simulink model "Simulator_Case_8"  (R2024a)
settings: Solver=VariableStepAuto  StartTime=0.0  StopTime=1400  RelTol=1e-3
values from neighbouring files (symbols this model uses):
  Declination_Sigean = 2.116*(pi/180)    (= 0.0369311669722)    [Parametrization_Simulation_Case_8.m]
  Position_Initial_X = Waypoints_X(1)    [Parametrization_Simulation_Case_8.m]
  Position_Initial_Y = Waypoints_Y(1)    [Parametrization_Simulation_Case_8.m]
  Time_Guidance_Sampling = 20    [Parametrization_Simulation_Case_8.m]
  Time_Period_Sampling = 0.1    [Parametrization_Simulation_Case_8.m]
  Velocity_Norm_Control_Vector = 0    [Velocity_Profile_Norm_Case_8.m]
undefined symbols (not defined in the file or in its folder): Area_Lateral_Projected_Wind, Damping_Coefficient, Damping_Factor_Waves, Density_Air, Density_Water_Salted, Draft_Depth, Drag_Coefficient, Gain_Filter, Inertia_Moment, Length_Ship, Longeron_Area, Mass_Ship, Pulsation_Natural, Pulsation_Wave, Rudder_Angle_Maximal, Rudder_Angle_Minimal, Rudder_Rate_Maximal, Rudder_Rate_Minimal, Static_Gain_Nomoto, Structure_Wind_Coefficient, Time_Constant_Total, Time_Stored, Velocity_Ship_Mean, Waypoints, Yaw_Control_Hydrodynamics_Derivative
libraries: simulink_extras x7, cstblocks x2, sensorinslib x2, sensorgpslib x1
(part 1 of 2)
settings Model: Creator=gerar  LastModifiedBy=gerar

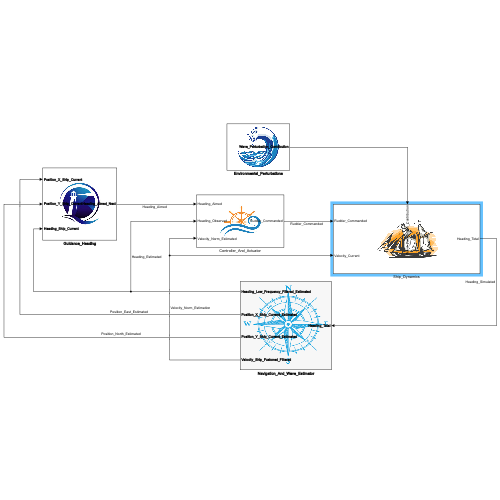
[thumbnail: Simulink's stored preview of the top-level diagram]
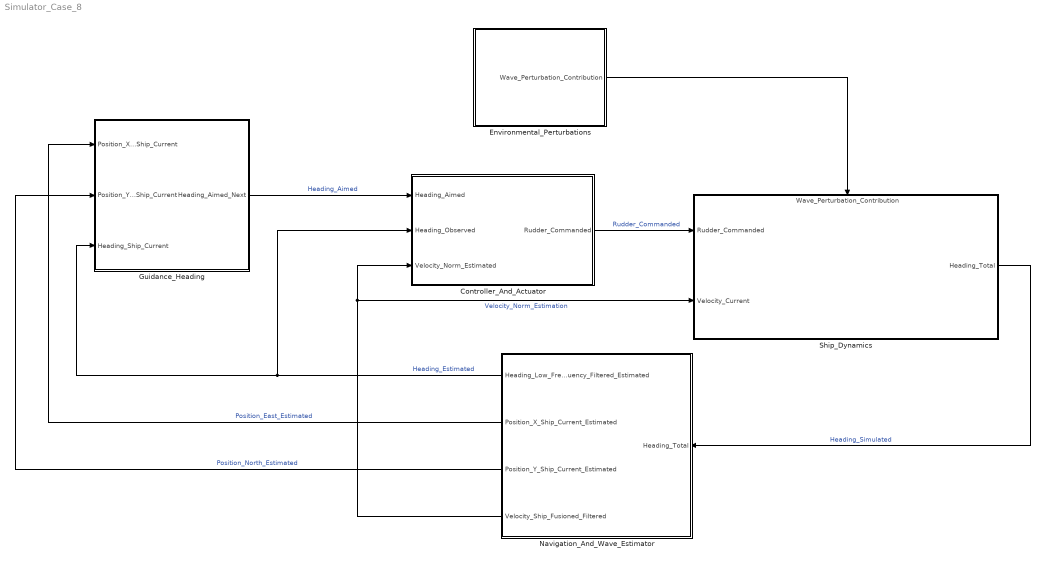
== system Simulator_Case_8 ==
  Controller_And_Actuator : Subsystem
      mask Display: image('Rudder3.jpg');
  Environmental_Perturbations : Subsystem
      mask Display: image('Wave2.png');
  Guidance_Heading : Subsystem
      mask Display: image('phare4.jpg');
  Navigation_And_Wave_Estimator : Subsystem
      mask Display: image('compass4.png');
  Ship_Dynamics : Subsystem
      settings: PortSchema="{\"entries\":[{\"content\":{\"sides\":[{\"content\":{\"connectorIds\":[\"In1\",\"In2\"]},\"type\":\"ConnectorPlacement.EquallySpacedRectSide\",\"uuid\":\"1262d93f-9737-49c5-b1c8-13d3f825160d\"},{\"content\":{\"connectorIds\":[\"Out1\"],\"side\":\"RIGHT\"},\"type\":\"ConnectorPlacement.EquallySpacedRectSide\",\"uuid\":\"2783823e-17f0-4da0-9b4a-e84aa912eb5f\"},{\"content\":{\"connectorIds\":[\"In3\"],\"side\":\"TOP\"},\"type\":\"ConnectorPlacement.EquallySpacedRectSide\",\"uuid\":\"9227960a-c500-4bd1-9392-f2e1de824969\"}]},\"type\":\"ConnectorPlacement.EquallySpacedConnector\",\"uuid\":\"fe1a7a14-057d-49da-982c-994c0d128614\"}],\"packageUris\":[\"http://schema.mathworks.com/mf0/Connector/R2020b\"],\"version\":\"1.0\"}"
      mask Display: image('ship2.png');
  wires:
  Guidance_Heading/1(Heading_Aimed_Next) -> Controller_And_Actuator/1(Heading_Aimed)  "Heading_Aimed"
  Navigation_And_Wave_Estimator/1(Heading_Low_Frequency_Filtered_Estimated) -> Controller_And_Actuator/2(Heading_Observed), Guidance_Heading/3(Heading_Ship_Current)  "Heading_Estimated"
  Environmental_Perturbations/1(Wave_Perturbation_Contribution) -> Ship_Dynamics/3(Wave_Perturbation_Contribution)
  Ship_Dynamics/1(Heading_Total) -> Navigation_And_Wave_Estimator/1(Heading_Total)  "Heading_Simulated"
  Navigation_And_Wave_Estimator/3(Position_Y_Ship_Current_Estimated) -> Guidance_Heading/2(Position_Y_Ship_Current)  "Position_North_Estimated"
  Navigation_And_Wave_Estimator/2(Position_X_Ship_Current_Estimated) -> Guidance_Heading/1(Position_X_Ship_Current)  "Position_East_Estimated"
  Controller_And_Actuator/1(Rudder_Commanded) -> Ship_Dynamics/1(Rudder_Commanded)  "Rudder_Commanded"
  Navigation_And_Wave_Estimator/4(Velocity_Ship_Fusioned_Filtered) -> Ship_Dynamics/2(Velocity_Current), Controller_And_Actuator/3(Velocity_Norm_Estimated)  "Velocity_Norm_Estimation"

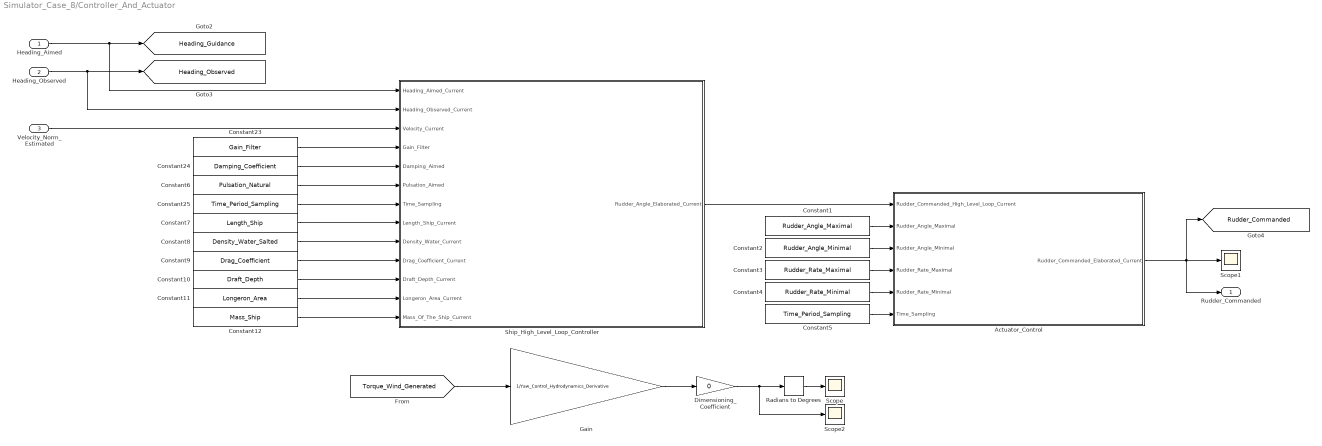
== system Simulator_Case_8/Controller_And_Actuator ==
  Heading_Aimed : Inport
  Heading_Observed : Inport  Port=2
  Velocity_Norm_Estimated : Inport  Port=3
  Actuator_Control : MATLAB Function  TreatAsAtomicUnit=on  SystemSampleTime=Time_Period_Sampling
  Constant1 : Constant  Value=Rudder_Angle_Maximal
  Constant10 : Constant  Value=Draft_Depth
  Constant11 : Constant  Value=Longeron_Area
  Constant12 : Constant  Value=Mass_Ship
  Constant2 : Constant  Value=Rudder_Angle_Minimal
  Constant23 : Constant  Value=Gain_Filter
  Constant24 : Constant  Value=Damping_Coefficient
  Constant25 : Constant  Value=Time_Period_Sampling
  Constant3 : Constant  Value=Rudder_Rate_Maximal
  Constant4 : Constant  Value=Rudder_Rate_Minimal
  Constant5 : Constant  Value=Time_Period_Sampling
  Constant6 : Constant  Value=Pulsation_Natural
  Constant7 : Constant  Value=Length_Ship
  Constant8 : Constant  Value=Density_Water_Salted
  Constant9 : Constant  Value=Drag_Coefficient
  Dimensioning_Coefficient : Gain  Gain=0
  Gain : Gain  Gain=1/Yaw_Control_Hydrodynamics_Derivative
  Radians to Degrees : simulink_extras/Transformations/Radians to Degrees
  Scope : Scope
  Scope1 : Scope
  Scope2 : Scope
  Ship_High_Level_Loop_Controller : MATLAB Function  TreatAsAtomicUnit=on  SystemSampleTime=Time_Period_Sampling
  Rudder_Commanded : Outport
  tag scope: Heading_Guidance=global, Heading_Observed=global, Rudder_Commanded=global
  wires:
  [Torque_Wind_Generated] -> Gain/1
  Gain/1 -> Dimensioning_Coefficient/1
  Radians to Degrees/1 -> Scope/1
  Dimensioning_Coefficient/1 -> Scope2/1, Radians to Degrees/1
  Heading_Aimed/1 -> [Heading_Guidance], Ship_High_Level_Loop_Controller/1(Heading_Aimed_Current)
  Heading_Observed/1 -> Ship_High_Level_Loop_Controller/2(Heading_Observed_Current), [Heading_Observed]
  Ship_High_Level_Loop_Controller/1(Rudder_Angle_Elaborated_Current) -> Actuator_Control/1(Rudder_Commanded_High_Level_Loop_Current)
  Constant1/1 -> Actuator_Control/2(Rudder_Angle_Maximal)
  Constant2/1 -> Actuator_Control/3(Rudder_Angle_Minimal)
  Constant3/1 -> Actuator_Control/4(Rudder_Rate_Maximal)
  Constant4/1 -> Actuator_Control/5(Rudder_Rate_Minimal)
  Constant5/1 -> Actuator_Control/6(Time_Sampling)
  Actuator_Control/1(Rudder_Commanded_Elaborated_Current) -> Rudder_Commanded/1, [Rudder_Commanded], Scope1/1
  Constant23/1 -> Ship_High_Level_Loop_Controller/4(Gain_Filter)
  Constant24/1 -> Ship_High_Level_Loop_Controller/5(Damping_Aimed)
  Constant25/1 -> Ship_High_Level_Loop_Controller/7(Time_Sampling)
  Constant6/1 -> Ship_High_Level_Loop_Controller/6(Pulsation_Aimed)
  Constant7/1 -> Ship_High_Level_Loop_Controller/8(Length_Ship_Current)
  Constant8/1 -> Ship_High_Level_Loop_Controller/9(Density_Water_Current)
  Constant9/1 -> Ship_High_Level_Loop_Controller/10(Drag_Coefficient_Current)
  Constant10/1 -> Ship_High_Level_Loop_Controller/11(Draft_Depth_Current)
  Constant11/1 -> Ship_High_Level_Loop_Controller/12(Longeron_Area_Current)
  Constant12/1 -> Ship_High_Level_Loop_Controller/13(Mass_Of_The_Ship_Current)
  Velocity_Norm_Estimated/1 -> Ship_High_Level_Loop_Controller/3(Velocity_Current)

== system Simulator_Case_8/Environmental_Perturbations ==
  Gain1 : Gain  Gain=0
  Scope : Scope
  Wave-Induced_Perturbation_Motion : Subsystem
  Wind_Perturbation_Torque : Subsystem
  Wave_Perturbation_Contribution : Outport
  tag scope: Torque_Wind_Generated=global, Wave_Generated_Signal=global
  wires:
  Wave-Induced_Perturbation_Motion/1(Wave_Induced_Heading) -> Scope/1, [Wave_Generated_Signal], Wave_Perturbation_Contribution/1
  Wind_Perturbation_Torque/1(Torque_Wind) -> Gain1/1
  Gain1/1 -> [Torque_Wind_Generated]

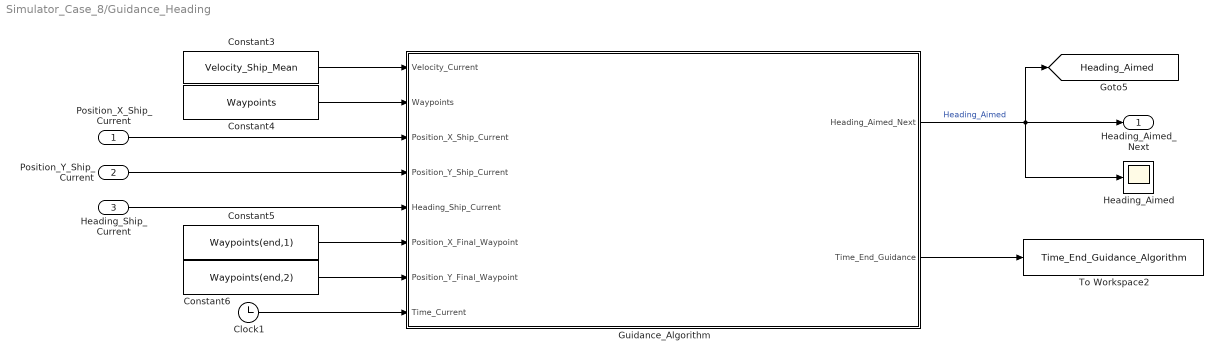
== system Simulator_Case_8/Guidance_Heading ==
  Position_X_Ship_Current : Inport
  Position_Y_Ship_Current : Inport  Port=2
  Heading_Ship_Current : Inport  Port=3
  Clock1 : Clock
  Constant3 : Constant  Value=Velocity_Ship_Mean
  Constant4 : Constant  Value=Waypoints
  Constant5 : Constant  Value=Waypoints(end,1)
  Constant6 : Constant  Value=Waypoints(end,2)
  Guidance_Algorithm : MATLAB Function  TreatAsAtomicUnit=on  SystemSampleTime=Time_Guidance_Sampling*3
  Heading_Aimed : Scope
  To Workspace2 : ToWorkspace  VariableName=Time_End_Guidance_Algorithm  SaveFormat=Timeseries  SampleTime=-1
  Heading_Aimed_Next : Outport
  tag scope: Heading_Aimed=global
  wires:
  Constant5/1 -> Guidance_Algorithm/6(Position_X_Final_Waypoint)
  Guidance_Algorithm/2(Time_End_Guidance) -> To Workspace2/1
  Constant3/1 -> Guidance_Algorithm/1(Velocity_Current)
  Position_Y_Ship_Current/1 -> Guidance_Algorithm/4(Position_Y_Ship_Current)
  Constant4/1 -> Guidance_Algorithm/2(Waypoints)
  Clock1/1 -> Guidance_Algorithm/8(Time_Current)
  Constant6/1 -> Guidance_Algorithm/7(Position_Y_Final_Waypoint)
  Position_X_Ship_Current/1 -> Guidance_Algorithm/3(Position_X_Ship_Current)
  Heading_Ship_Current/1 -> Guidance_Algorithm/5(Heading_Ship_Current)
  Guidance_Algorithm/1(Heading_Aimed_Next) -> Heading_Aimed/1, Heading_Aimed_Next/1, [Heading_Aimed]  "Heading_Aimed"

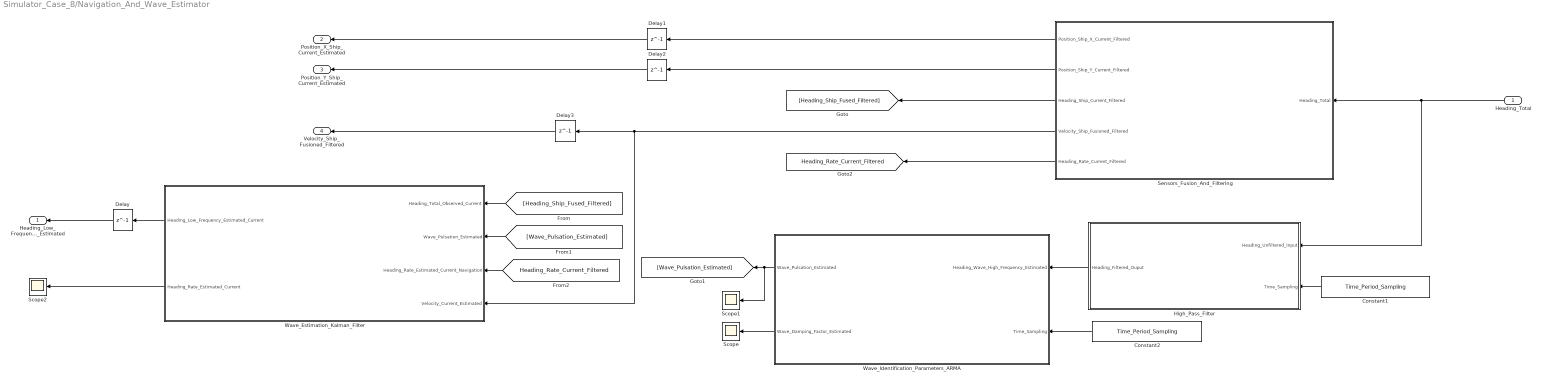
== system Simulator_Case_8/Navigation_And_Wave_Estimator ==
  Heading_Total : Inport
  Constant1 : Constant  Value=Time_Period_Sampling
  Constant2 : Constant  Value=Time_Period_Sampling
  Delay{,1..3} (4 alike) : Delay  DelayLength=1  InputProcessing=Columns as channels (frame based)  SampleTime=Time_Period_Sampling
  High_Pass_Filter : MATLAB Function  TreatAsAtomicUnit=on  SystemSampleTime=Time_Period_Sampling
  Scope : Scope
  Scope1 : Scope
  Scope2 : Scope
  Sensors_Fusion_And_Filtering : Subsystem
  Wave_Estimation_Kalman_Filter : Subsystem
  Wave_Identification_Parameters_ARMA : MATLAB Function  TreatAsAtomicUnit=on  SystemSampleTime=Time_Period_Sampling
  Heading_Low_Frequency_Filtered_Estimated : Outport
  Position_X_Ship_Current_Estimated : Outport  Port=2
  Position_Y_Ship_Current_Estimated : Outport  Port=3
  Velocity_Ship_Fusioned_Filtered : Outport  Port=4
  tag scope: Heading_Rate_Current_Filtered=global
  wires:
  Delay1/1 -> Position_X_Ship_Current_Estimated/1
  Delay2/1 -> Position_Y_Ship_Current_Estimated/1
  Sensors_Fusion_And_Filtering/1(Position_Ship_X_Current_Filtered) -> Delay1/1
  Sensors_Fusion_And_Filtering/2(Position_Ship_Y_Current_Filtered) -> Delay2/1
  Wave_Estimation_Kalman_Filter/1(Heading_Low_Frequency_Estimated_Current) -> Delay/1
  High_Pass_Filter/1(Heading_Filtered_Ouput) -> Wave_Identification_Parameters_ARMA/1(Heading_Wave_High_Frequency_Estimated)
  Constant1/1 -> High_Pass_Filter/2(Time_Sampling)
  Heading_Total/1 -> High_Pass_Filter/1(Heading_Unfiltered_Input), Sensors_Fusion_And_Filtering/1(Heading_Total)
  Delay/1 -> Heading_Low_Frequency_Filtered_Estimated/1
  Wave_Estimation_Kalman_Filter/2(Heading_Rate_Estimated_Current) -> Scope2/1
  Constant2/1 -> Wave_Identification_Parameters_ARMA/2(Time_Sampling)
  Sensors_Fusion_And_Filtering/3(Heading_Ship_Current_Filtered) -> [Heading_Ship_Fused_Filtered]
  [Heading_Ship_Fused_Filtered] -> Wave_Estimation_Kalman_Filter/1(Heading_Total_Observed_Current)
  Wave_Identification_Parameters_ARMA/1(Wave_Pulsation_Estimated) -> Scope1/1, [Wave_Pulsation_Estimated]
  [Wave_Pulsation_Estimated] -> Wave_Estimation_Kalman_Filter/2(Wave_Pulsation_Estimated)
  Wave_Identification_Parameters_ARMA/2(Wave_Damping_Factor_Estimated) -> Scope/1
  Sensors_Fusion_And_Filtering/4(Velocity_Ship_Fusioned_Filtered) -> Wave_Estimation_Kalman_Filter/4(Velocity_Current_Estimated), Delay3/1
  Delay3/1 -> Velocity_Ship_Fusioned_Filtered/1
  Sensors_Fusion_And_Filtering/5(Heading_Rate_Current_Filtered) -> [Heading_Rate_Current_Filtered]
  [Heading_Rate_Current_Filtered] -> Wave_Estimation_Kalman_Filter/3(Heading_Rate_Estimated_Current_Navigation)

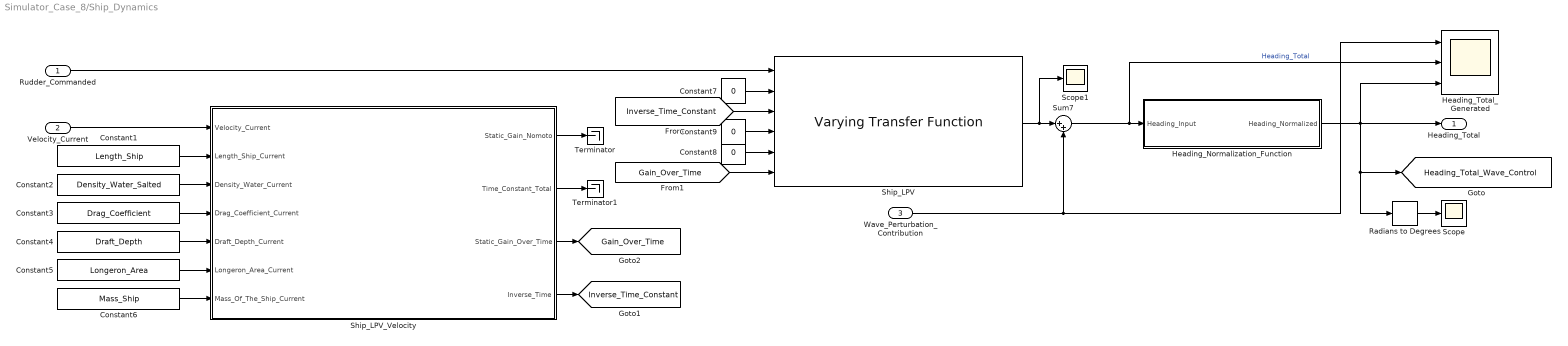
== system Simulator_Case_8/Ship_Dynamics ==
  Rudder_Commanded : Inport
  Velocity_Current : Inport  Port=2
  Wave_Perturbation_Contribution : Inport  Port=3
  Constant1 : Constant  Value=Length_Ship
  Constant2 : Constant  Value=Density_Water_Salted
  Constant3 : Constant  Value=Drag_Coefficient
  Constant4 : Constant  Value=Draft_Depth
  Constant5 : Constant  Value=Longeron_Area
  Constant6 : Constant  Value=Mass_Ship
  Constant7 : Constant  Value=0
  Constant8 : Constant  Value=0
  Constant9 : Constant  Value=0
  Heading_Normalization_Function : MATLAB Function  TreatAsAtomicUnit=on
  Heading_Total_Generated : Scope  NumInputPorts=3
  Radians to Degrees : simulink_extras/Transformations/Radians to Degrees
  Scope : Scope
  Scope1 : Scope
  Ship_LPV : cstblocks/Linear Parameter Varying/Varying Transfer Function  N=2  Feedthrough=on
  Ship_LPV_Velocity : MATLAB Function  TreatAsAtomicUnit=on
  Sum7 : Sum  Inputs=|++
  Terminator : Terminator
  Terminator1 : Terminator
  Heading_Total : Outport
  tag scope: Gain_Over_Time=global, Heading_Total_Wave_Control=global, Inverse_Time_Constant=global
  wires:
  Ship_LPV/1 -> Scope1/1, Sum7/1
  Wave_Perturbation_Contribution/1 -> Sum7/2, Heading_Total_Generated/1
  Sum7/1 -> Heading_Total_Generated/2, Heading_Normalization_Function/1(Heading_Input)  "Heading_Total"
  Radians to Degrees/1 -> Scope/1
  Heading_Normalization_Function/1(Heading_Normalized) -> Radians to Degrees/1, [Heading_Total_Wave_Control], Heading_Total_Generated/3, Heading_Total/1
  Constant1/1 -> Ship_LPV_Velocity/2(Length_Ship_Current)
  Constant3/1 -> Ship_LPV_Velocity/4(Drag_Coefficient_Current)
  Constant6/1 -> Ship_LPV_Velocity/7(Mass_Of_The_Ship_Current)
  Constant4/1 -> Ship_LPV_Velocity/5(Draft_Depth_Current)
  Constant2/1 -> Ship_LPV_Velocity/3(Density_Water_Current)
  Velocity_Current/1 -> Ship_LPV_Velocity/1(Velocity_Current)
  Constant5/1 -> Ship_LPV_Velocity/6(Longeron_Area_Current)
  Constant7/1 -> Ship_LPV/2
  Constant9/1 -> Ship_LPV/4
  Constant8/1 -> Ship_LPV/5
  Rudder_Commanded/1 -> Ship_LPV/1
  Ship_LPV_Velocity/4(Inverse_Time) -> [Inverse_Time_Constant]
  [Inverse_Time_Constant] -> Ship_LPV/3
  Ship_LPV_Velocity/3(Static_Gain_Over_Time) -> [Gain_Over_Time]
  [Gain_Over_Time] -> Ship_LPV/6
  Ship_LPV_Velocity/1(Static_Gain_Nomoto) -> Terminator/1
  Ship_LPV_Velocity/2(Time_Constant_Total) -> Terminator1/1

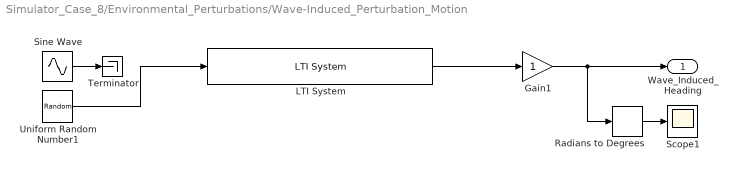
== system Simulator_Case_8/Environmental_Perturbations/Wave-Induced_Perturbation_Motion ==
  Gain1 : Gain
  LTI System : cstblocks/LTI System  sys=Wave_Transfer_Function  IC=[]  PadeOrder=0
  Radians to Degrees : simulink_extras/Transformations/Radians to Degrees
  Scope1 : Scope
  Sine Wave : Sin  Amplitude=2*(pi/180)  Frequency=Pulsation_Wave  SampleTime=0
  Terminator : Terminator
  Uniform Random Number1 : UniformRandomNumber  Minimum=-10*(pi/180)  Maximum=10*(pi/180)  SampleTime=Time_Period_Sampling
  Wave_Induced_Heading : Outport
  wires:
  Radians to Degrees/1 -> Scope1/1
  LTI System/1 -> Gain1/1
  Gain1/1 -> Radians to Degrees/1, Wave_Induced_Heading/1
  Uniform Random Number1/1 -> LTI System/1
  Sine Wave/1 -> Terminator/1

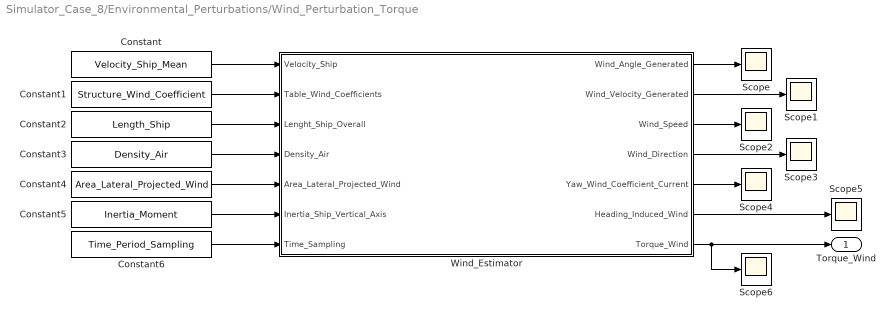
== system Simulator_Case_8/Environmental_Perturbations/Wind_Perturbation_Torque ==
  Constant : Constant  Value=Velocity_Ship_Mean
  Constant1 : Constant  Value=Structure_Wind_Coefficient
  Constant2 : Constant  Value=Length_Ship
  Constant3 : Constant  Value=Density_Air
  Constant4 : Constant  Value=Area_Lateral_Projected_Wind
  Constant5 : Constant  Value=Inertia_Moment
  Constant6 : Constant  Value=Time_Period_Sampling
  Scope{,1..6} (7 alike) : Scope
  Wind_Estimator : MATLAB Function  TreatAsAtomicUnit=on  SystemSampleTime=Time_Period_Sampling
  Torque_Wind : Outport
  wires:
  Wind_Estimator/5(Yaw_Wind_Coefficient_Current) -> Scope4/1
  Constant2/1 -> Wind_Estimator/3(Lenght_Ship_Overall)
  Constant/1 -> Wind_Estimator/1(Velocity_Ship)
  Constant5/1 -> Wind_Estimator/6(Inertia_Ship_Vertical_Axis)
  Constant4/1 -> Wind_Estimator/5(Area_Lateral_Projected_Wind)
  Constant3/1 -> Wind_Estimator/4(Density_Air)
  Wind_Estimator/1(Wind_Angle_Generated) -> Scope/1
  Wind_Estimator/2(Wind_Velocity_Generated) -> Scope1/1
  Wind_Estimator/3(Wind_Speed) -> Scope2/1
  Wind_Estimator/7(Torque_Wind) -> Torque_Wind/1, Scope6/1
  Constant1/1 -> Wind_Estimator/2(Table_Wind_Coefficients)
  Constant6/1 -> Wind_Estimator/7(Time_Sampling)
  Wind_Estimator/6(Heading_Induced_Wind) -> Scope5/1
  Wind_Estimator/4(Wind_Direction) -> Scope3/1

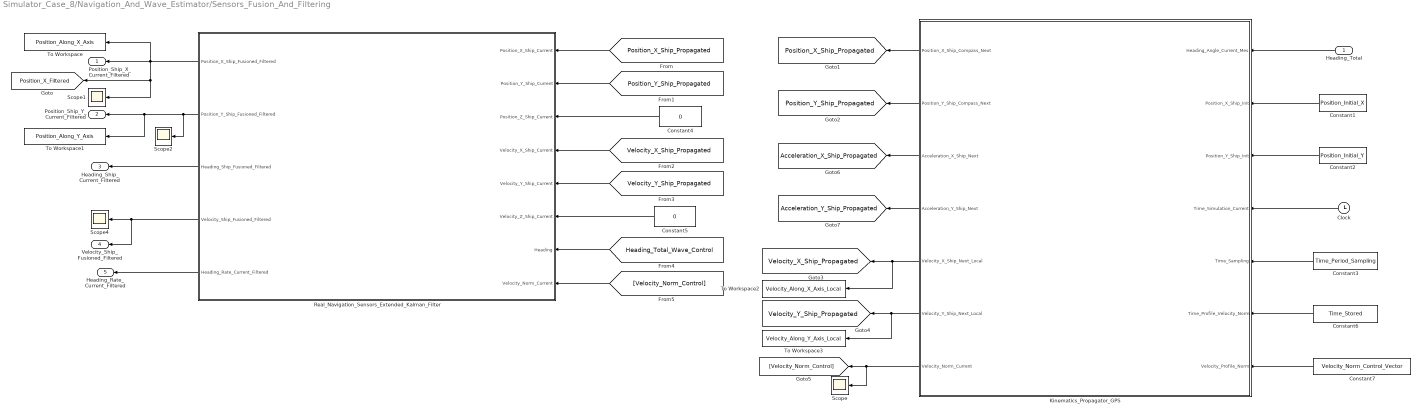
== system Simulator_Case_8/Navigation_And_Wave_Estimator/Sensors_Fusion_And_Filtering ==
  Heading_Total : Inport
  Clock : Clock
  Constant1 : Constant  Value=Position_Initial_X
  Constant2 : Constant  Value=Position_Initial_Y
  Constant3 : Constant  Value=Time_Period_Sampling
  Constant4 : Constant  Value=0
  Constant5 : Constant  Value=0
  Constant6 : Constant  Value=Time_Stored
  Constant7 : Constant  Value=Velocity_Norm_Control_Vector
  Kinematics_Propagator_GPS : MATLAB Function  TreatAsAtomicUnit=on  SystemSampleTime=Time_Period_Sampling
  Real_Navigation_Sensors_Extended_Kalman_Filter : Subsystem
  Scope{,1..2,4} (4 alike) : Scope
  To Workspace : ToWorkspace  VariableName=Position_Along_X_Axis  SaveFormat=Timeseries  SampleTime=Time_Period_Sampling
  To Workspace1 : ToWorkspace  VariableName=Position_Along_Y_Axis  SaveFormat=Timeseries  SampleTime=Time_Period_Sampling
  To Workspace2 : ToWorkspace  VariableName=Velocity_Along_X_Axis_Local  SaveFormat=Timeseries  SampleTime=Time_Period_Sampling
  To Workspace3 : ToWorkspace  VariableName=Velocity_Along_Y_Axis_Local  SaveFormat=Timeseries  SampleTime=Time_Period_Sampling
  Position_Ship_X_Current_Filtered : Outport
  Position_Ship_Y_Current_Filtered : Outport  Port=2
  Heading_Ship_Current_Filtered : Outport  Port=3
  Velocity_Ship_Fusioned_Filtered : Outport  Port=4
  Heading_Rate_Current_Filtered : Outport  Port=5
  tag scope: Acceleration_X_Ship_Propagated=global, Acceleration_Y_Ship_Propagated=global, Position_X_Filtered=global, Position_X_Ship_Propagated=global, Position_Y_Ship_Propagated=global, Velocity_X_Ship_Propagated=global, Velocity_Y_Ship_Propagated=global
  wires:
  Constant2/1 -> Kinematics_Propagator_GPS/3(Position_Y_Ship_Init)
  Clock/1 -> Kinematics_Propagator_GPS/4(Time_Simulation_Current)
  Constant1/1 -> Kinematics_Propagator_GPS/2(Position_X_Ship_Init)
  Constant3/1 -> Kinematics_Propagator_GPS/5(Time_Sampling)
  Kinematics_Propagator_GPS/3(Acceleration_X_Ship_Next) -> [Acceleration_X_Ship_Propagated]
  Kinematics_Propagator_GPS/4(Acceleration_Y_Ship_Next) -> [Acceleration_Y_Ship_Propagated]
  Heading_Total/1 -> Kinematics_Propagator_GPS/1(Heading_Angle_Current_Mes)
  Kinematics_Propagator_GPS/5(Velocity_X_Ship_Next_Local) -> To Workspace2/1, [Velocity_X_Ship_Propagated]
  Kinematics_Propagator_GPS/6(Velocity_Y_Ship_Next_Local) -> To Workspace3/1, [Velocity_Y_Ship_Propagated]
  Kinematics_Propagator_GPS/1(Position_X_Ship_Compass_Next) -> [Position_X_Ship_Propagated]
  Kinematics_Propagator_GPS/2(Position_Y_Ship_Compass_Next) -> [Position_Y_Ship_Propagated]
  [Position_X_Ship_Propagated] -> Real_Navigation_Sensors_Extended_Kalman_Filter/1(Position_X_Ship_Current)
  [Position_Y_Ship_Propagated] -> Real_Navigation_Sensors_Extended_Kalman_Filter/2(Position_Y_Ship_Current)
  Constant4/1 -> Real_Navigation_Sensors_Extended_Kalman_Filter/3(Position_Z_Ship_Current)
  [Velocity_X_Ship_Propagated] -> Real_Navigation_Sensors_Extended_Kalman_Filter/4(Velocity_X_Ship_Current)
  [Velocity_Y_Ship_Propagated] -> Real_Navigation_Sensors_Extended_Kalman_Filter/5(Velocity_Y_Ship_Current)
  Constant5/1 -> Real_Navigation_Sensors_Extended_Kalman_Filter/6(Velocity_Z_Ship_Current)
  [Heading_Total_Wave_Control] -> Real_Navigation_Sensors_Extended_Kalman_Filter/7(Heading)
  Real_Navigation_Sensors_Extended_Kalman_Filter/1(Position_X_Ship_Fusioned_Filtered) -> Scope1/1, [Position_X_Filtered], Position_Ship_X_Current_Filtered/1, To Workspace/1
  Real_Navigation_Sensors_Extended_Kalman_Filter/2(Position_Y_Ship_Fusioned_Filtered) -> Scope2/1, To Workspace1/1, Position_Ship_Y_Current_Filtered/1
  Real_Navigation_Sensors_Extended_Kalman_Filter/3(Heading_Ship_Fusioned_Filtered) -> Heading_Ship_Current_Filtered/1
  Real_Navigation_Sensors_Extended_Kalman_Filter/4(Velocity_Ship_Fusioned_Filtered) -> Velocity_Ship_Fusioned_Filtered/1, Scope4/1
  Kinematics_Propagator_GPS/7(Velocity_Norm_Current) -> Scope/1, [Velocity_Norm_Control]
  Constant6/1 -> Kinematics_Propagator_GPS/6(Time_Profile_Velocity_Norm)
  Constant7/1 -> Kinematics_Propagator_GPS/7(Velocity_Profile_Norm)
  [Velocity_Norm_Control] -> Real_Navigation_Sensors_Extended_Kalman_Filter/8(Velocity_Norm_Current)
  Real_Navigation_Sensors_Extended_Kalman_Filter/5(Heading_Rate_Current_Filtered) -> Heading_Rate_Current_Filtered/1

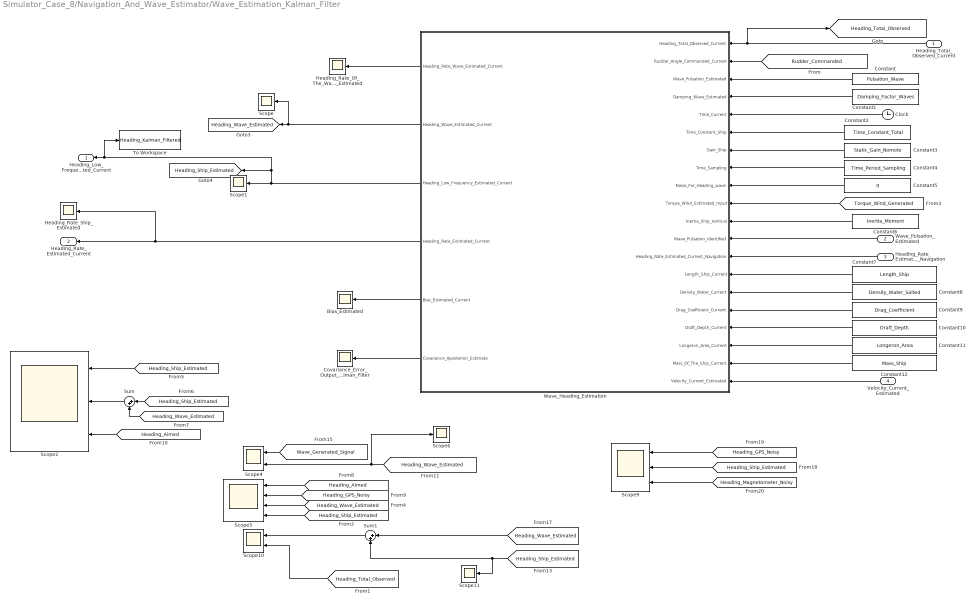
== system Simulator_Case_8/Navigation_And_Wave_Estimator/Wave_Estimation_Kalman_Filter ==
  Heading_Total_Observed_Current : Inport
  Wave_Pulsation_Estimated : Inport  Port=2
  Heading_Rate_Estimated_Current_Navigation : Inport  Port=3
  Velocity_Current_Estimated : Inport  Port=4
  Bias_Estimated : Scope
  Clock : Clock
  Constant : Constant  Value=Pulsation_Wave  SampleTime=Time_Period_Sampling
  Constant1 : Constant  Value=Damping_Factor_Waves  SampleTime=Time_Period_Sampling
  Constant10 : Constant  Value=Draft_Depth
  Constant11 : Constant  Value=Longeron_Area
  Constant12 : Constant  Value=Mass_Ship
  Constant2 : Constant  Value=Time_Constant_Total  SampleTime=Time_Period_Sampling
  Constant3 : Constant  Value=Static_Gain_Nomoto  SampleTime=Time_Period_Sampling
  Constant4 : Constant  Value=Time_Period_Sampling  SampleTime=Time_Period_Sampling
  Constant5 : Constant  Value=0
  Constant6 : Constant  Value=Inertia_Moment
  Constant7 : Constant  Value=Length_Ship
  Constant8 : Constant  Value=Density_Water_Salted
  Constant9 : Constant  Value=Drag_Coefficient
  Covariance_Error_Output_Kalman_Filter : Scope
  Heading_Rate_Of_The_Waves_Estimated : Scope
  Heading_Rate_Ship_Estimated : Scope
  Scope{,1,6,11} (4 alike) : Scope
  Scope10 : Scope  NumInputPorts=2
  Scope2 : Scope  NumInputPorts=3
  Scope4 : Scope  NumInputPorts=2
  Scope5 : Scope  NumInputPorts=4
  Scope9 : Scope  NumInputPorts=3
  Sum : Sum  Inputs=|++
  Sum1 : Sum  Inputs=|++
  To Workspace : ToWorkspace  VariableName=Heading_Kalman_Filtered  SaveFormat=Timeseries  SampleTime=Time_Period_Sampling
  Wave_Heading_Estimation : MATLAB Function  TreatAsAtomicUnit=on  SystemSampleTime=Time_Period_Sampling
  Heading_Low_Frequency_Estimated_Current : Outport
  Heading_Rate_Estimated_Current : Outport  Port=2
  tag scope: Heading_Ship_Estimated=global, Heading_Total_Observed=global, Heading_Wave_Estimated=global
  wires:
  Wave_Heading_Estimation/3(Heading_Low_Frequency_Estimated_Current) -> To Workspace/1, Heading_Low_Frequency_Estimated_Current/1, [Heading_Ship_Estimated], Scope1/1
  Heading_Total_Observed_Current/1 -> [Heading_Total_Observed], Wave_Heading_Estimation/1(Heading_Total_Observed_Current)
  [Rudder_Commanded] -> Wave_Heading_Estimation/2(Rudder_Angle_Commanded_Current)
  Constant/1 -> Wave_Heading_Estimation/3(Wave_Pulsation_Estimated)
  Constant1/1 -> Wave_Heading_Estimation/4(Damping_Wave_Estimated)
  Clock/1 -> Wave_Heading_Estimation/5(Time_Current)
  Constant2/1 -> Wave_Heading_Estimation/6(Time_Constant_Ship)
  Constant3/1 -> Wave_Heading_Estimation/7(Gain_Ship)
  Constant4/1 -> Wave_Heading_Estimation/8(Time_Sampling)
  Constant5/1 -> Wave_Heading_Estimation/9(Noise_For_Heading_wave)
  Wave_Heading_Estimation/1(Heading_Rate_Wave_Estimated_Current) -> Heading_Rate_Of_The_Waves_Estimated/1
  Wave_Heading_Estimation/2(Heading_Wave_Estimated_Current) -> Scope/1, [Heading_Wave_Estimated]
  Wave_Heading_Estimation/5(Bias_Estimated_Current) -> Bias_Estimated/1
  Wave_Heading_Estimation/4(Heading_Rate_Estimated_Current) -> Heading_Rate_Ship_Estimated/1, Heading_Rate_Estimated_Current/1
  Wave_Heading_Estimation/6(Covariance_Aposteriori_Estimate) -> Covariance_Error_Output_Kalman_Filter/1
  [Heading_Aimed] -> Scope5/1
  [Wave_Generated_Signal] -> Scope4/1
  [Heading_Ship_Estimated] -> Scope9/2
  [Heading_Magnetometer_Noisy] -> Scope9/3
  [Heading_Ship_Estimated] -> Scope11/1, Sum1/2
  [Heading_GPS_Noisy] -> Scope9/1
  [Heading_Wave_Estimated] -> Sum1/1
  Sum1/1 -> Scope10/1
  [Heading_GPS_Noisy] -> Scope5/2
  [Heading_Ship_Estimated] -> Scope5/4
  [Heading_Wave_Estimated] -> Scope6/1, Scope4/2
  [Heading_Total_Observed] -> Scope10/2
  Constant6/1 -> Wave_Heading_Estimation/11(Inertia_Ship_Vertical)
  [Torque_Wind_Generated] -> Wave_Heading_Estimation/10(Torque_Wind_Estimated_Input)
  Wave_Pulsation_Estimated/1 -> Wave_Heading_Estimation/12(Wave_Pulsation_Identified)
  Heading_Rate_Estimated_Current_Navigation/1 -> Wave_Heading_Estimation/13(Heading_Rate_Estimated_Current_Navigation)
  Constant7/1 -> Wave_Heading_Estimation/14(Length_Ship_Current)
  Constant8/1 -> Wave_Heading_Estimation/15(Density_Water_Current)
  [Heading_Wave_Estimated] -> Scope5/3
  [Heading_Ship_Estimated] -> Scope2/1
  Sum/1 -> Scope2/2
  [Heading_Ship_Estimated] -> Sum/1
  [Heading_Wave_Estimated] -> Sum/2
  [Heading_Aimed] -> Scope2/3
  Constant9/1 -> Wave_Heading_Estimation/16(Drag_Coefficient_Current)
  Constant10/1 -> Wave_Heading_Estimation/17(Draft_Depth_Current)
  Constant11/1 -> Wave_Heading_Estimation/18(Longeron_Area_Current)
  Constant12/1 -> Wave_Heading_Estimation/19(Mass_Of_The_Ship_Current)
  Velocity_Current_Estimated/1 -> Wave_Heading_Estimation/20(Velocity_Current_Estimated)

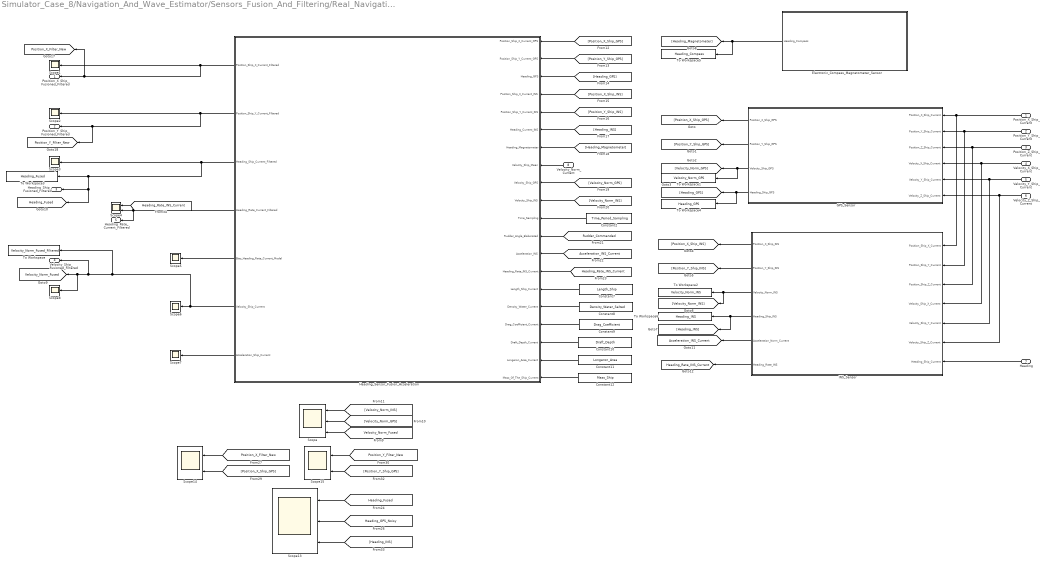
== system Simulator_Case_8/Navigation_And_Wave_Estimator/Sensors_Fusion_And_Filtering/Real_Navigation_Sensors_Extended_Kalman_Filter ==
  Position_X_Ship_Current : Inport
  Position_Y_Ship_Current : Inport  Port=2
  Position_Z_Ship_Current : Inport  Port=3
  Velocity_X_Ship_Current : Inport  Port=4
  Velocity_Y_Ship_Current : Inport  Port=5
  Velocity_Z_Ship_Current : Inport  Port=6
  Heading : Inport  Port=7
  Velocity_Norm_Current : Inport  Port=8
  Constant10 : Constant  Value=Draft_Depth
  Constant11 : Constant  Value=Longeron_Area
  Constant12 : Constant  Value=Mass_Ship
  Constant2 : Constant  Value=Time_Period_Sampling
  Constant7 : Constant  Value=Length_Ship
  Constant8 : Constant  Value=Density_Water_Salted
  Constant9 : Constant  Value=Drag_Coefficient
  Electronic_Compass_Magnetometer_Sensor : Subsystem
  GPS_Sensor : Subsystem
  Heading_Sensor_Fusion_Acceleration : MATLAB Function  TreatAsAtomicUnit=on  SystemSampleTime=Time_Period_Sampling
  INS_Sensor : Subsystem
  Scope : Scope  NumInputPorts=3
  Scope{1..3,5..8} (7 alike) : Scope
  Scope13 : Scope  NumInputPorts=3
  Scope14 : Scope  NumInputPorts=2
  Scope15 : Scope  NumInputPorts=2
  Scope4 : Scope  NumInputPorts=2
  To Workspace : ToWorkspace  VariableName=Velocity_Norm_Fused_Filtered  SaveFormat=Timeseries  SampleTime=-1
  To Workspace1 : ToWorkspace  VariableName=Velocity_Norm_GPS  SaveFormat=Timeseries  SampleTime=-1
  To Workspace2 : ToWorkspace  VariableName=Velocity_Norm_INS  SaveFormat=Timeseries  SampleTime=-1
  To Workspace3 : ToWorkspace  VariableName=Heading_Fused  SaveFormat=Timeseries  SampleTime=-1
  To Workspace4 : ToWorkspace  VariableName=Heading_GPS  SaveFormat=Timeseries  SampleTime=-1
  To Workspace5 : ToWorkspace  VariableName=Heading_Compass  SaveFormat=Timeseries  SampleTime=-1
  To Workspace6 : ToWorkspace  VariableName=Heading_INS  SaveFormat=Timeseries  SampleTime=-1
  Position_X_Ship_Fusioned_Filtered : Outport
  Position_Y_Ship_Fusioned_Filtered : Outport  Port=2
  Heading_Ship_Fusioned_Filtered : Outport  Port=3
  Velocity_Ship_Fusioned_Filtered : Outport  Port=4
  Heading_Rate_Current_Filtered : Outport  Port=5
  tag scope: Acceleration_INS_Current=global, Heading_Fused=global, Heading_Rate_INS_Current=global, Position_X_Filter_New=global, Position_Y_Filter_New=global, Velocity_Norm_Fused=global
  wires:
  Electronic_Compass_Magnetometer_Sensor/1(Heading_Compass) -> To Workspace5/1, [Heading_Magnetometer]
  Position_Z_Ship_Current/1 -> INS_Sensor/3(Position_Ship_Z_Current), GPS_Sensor/3(Position_Z_Ship_Current)
  Velocity_Z_Ship_Current/1 -> INS_Sensor/6(Velocity_Ship_Z_Current), GPS_Sensor/6(Velocity_Z_Ship_Current)
  GPS_Sensor/1(Position_X_Ship_GPS) -> [Position_X_Ship_GPS]
  GPS_Sensor/2(Position_Y_Ship_GPS) -> [Position_Y_Ship_GPS]
  GPS_Sensor/3(Velocity_Ship_GPS) -> To Workspace1/1, [Velocity_Norm_GPS]
  GPS_Sensor/4(Heading_Ship_GPS) -> To Workspace4/1, [Heading_GPS]
  Position_X_Ship_Current/1 -> INS_Sensor/1(Position_Ship_X_Current), GPS_Sensor/1(Position_X_Ship_Current)
  Velocity_X_Ship_Current/1 -> INS_Sensor/4(Velocity_Ship_X_Current), GPS_Sensor/4(Velocity_X_Ship_Current)
  Velocity_Y_Ship_Current/1 -> INS_Sensor/5(Velocity_Ship_Y_Current), GPS_Sensor/5(Velocity_Y_Ship_Current)
  Position_Y_Ship_Current/1 -> INS_Sensor/2(Position_Ship_Y_Current), GPS_Sensor/2(Position_Y_Ship_Current)
  INS_Sensor/1(Position_X_Ship_INS) -> [Position_X_Ship_INS]
  INS_Sensor/2(Position_Y_Ship_INS) -> [Position_Y_Ship_INS]
  INS_Sensor/3(Velocity_Norm_INS) -> [Velocity_Norm_INS], To Workspace2/1
  INS_Sensor/4(Heading_Ship_INS) -> [Heading_INS], To Workspace6/1
  [Velocity_Norm_Fused] -> Scope/3
  [Velocity_Norm_GPS] -> Scope/2
  [Velocity_Norm_INS] -> Scope/1
  Velocity_Norm_Current/1 -> Heading_Sensor_Fusion_Acceleration/8(Velocity_Ship_Mean)
  [Heading_INS] -> Heading_Sensor_Fusion_Acceleration/6(Heading_Current_INS)
  [Heading_Magnetometer] -> Heading_Sensor_Fusion_Acceleration/7(Heading_Magnetometer)
  [Heading_GPS] -> Heading_Sensor_Fusion_Acceleration/3(Heading_GPS)
  [Velocity_Norm_INS] -> Heading_Sensor_Fusion_Acceleration/10(Velocity_Ship_INS)
  [Position_X_Ship_INS] -> Heading_Sensor_Fusion_Acceleration/4(Position_Ship_X_Current_INS)
  [Position_Y_Ship_INS] -> Heading_Sensor_Fusion_Acceleration/5(Position_Ship_Y_Current_INS)
  [Velocity_Norm_GPS] -> Heading_Sensor_Fusion_Acceleration/9(Velocity_Ship_GPS)
  [Position_Y_Ship_GPS] -> Heading_Sensor_Fusion_Acceleration/2(Position_Ship_Y_Current_GPS)
  Constant2/1 -> Heading_Sensor_Fusion_Acceleration/11(Time_Sampling)
  [Position_X_Ship_GPS] -> Heading_Sensor_Fusion_Acceleration/1(Position_Ship_X_Current_GPS)
  Heading_Sensor_Fusion_Acceleration/1(Position_Ship_X_Current_Filtered) -> [Position_X_Filter_New], Position_X_Ship_Fusioned_Filtered/1, Scope1/1
  Heading_Sensor_Fusion_Acceleration/2(Position_Ship_Y_Current_Filtered) -> [Position_Y_Filter_New], Position_Y_Ship_Fusioned_Filtered/1, Scope2/1
  Heading_Sensor_Fusion_Acceleration/3(Heading_Ship_Current_Filtered) -> Heading_Ship_Fusioned_Filtered/1, [Heading_Fused], To Workspace3/1, Scope3/1
  Heading_Sensor_Fusion_Acceleration/4(Heading_Rate_Current_Filtered) -> Heading_Rate_Current_Filtered/1, Scope4/2
  [Rudder_Commanded] -> Heading_Sensor_Fusion_Acceleration/12(Rudder_Angle_Elaborated)
  Heading_Sensor_Fusion_Acceleration/5(Bias_Heading_Rate_Current_Model) -> Scope5/1
  Heading/1 -> INS_Sensor/7(Heading_Ship_Current)
  INS_Sensor/5(Acceleration_Norm_Current) -> [Acceleration_INS_Current]
  [Acceleration_INS_Current] -> Heading_Sensor_Fusion_Acceleration/13(Acceleration_INS)
  Heading_Sensor_Fusion_Acceleration/6(Velocity_Ship_Current) -> To Workspace/1, Velocity_Ship_Fusioned_Filtered/1, Scope8/1, [Velocity_Norm_Fused], Scope6/1
  Heading_Sensor_Fusion_Acceleration/7(Acceleration_Ship_Current) -> Scope7/1
  INS_Sensor/6(Heading_Rate_INS) -> [Heading_Rate_INS_Current]
  [Heading_Rate_INS_Current] -> Heading_Sensor_Fusion_Acceleration/14(Heading_Rate_INS_Current)
  Constant12/1 -> Heading_Sensor_Fusion_Acceleration/20(Mass_Of_The_Ship_Current)
  Constant11/1 -> Heading_Sensor_Fusion_Acceleration/19(Longeron_Area_Current)
  Constant10/1 -> Heading_Sensor_Fusion_Acceleration/18(Draft_Depth_Current)
  Constant9/1 -> Heading_Sensor_Fusion_Acceleration/17(Drag_Coefficient_Current)
  Constant8/1 -> Heading_Sensor_Fusion_Acceleration/16(Density_Water_Current)
  Constant7/1 -> Heading_Sensor_Fusion_Acceleration/15(Length_Ship_Current)
  [Heading_GPS_Noisy] -> Scope13/2
  [Heading_Fused] -> Scope13/1
  [Position_X_Filter_New] -> Scope14/1
  [Position_X_Ship_GPS] -> Scope14/2
  [Position_Y_Filter_New] -> Scope15/1
  [Position_Y_Ship_GPS] -> Scope15/2
  [Heading_INS] -> Scope13/3
  [Heading_Rate_INS_Current] -> Scope4/1

== system Simulator_Case_8/Navigation_And_Wave_Estimator/Sensors_Fusion_And_Filtering/Real_Navigation_Sensors_Extended_Kalman_Filter/Electronic_Compass_Magnetometer_Sensor ==
  Constant : Constant  Value=Declination_Sigean
  Scope8 : Scope
  Sum : Sum  Inputs=|++
  To Workspace1 : ToWorkspace  VariableName=Heading_Noisy_Magnetometer  SaveFormat=Timeseries  SampleTime=Time_Period_Sampling
  Heading_Compass : Outport
  tag scope: Heading_Magnetometer_Noisy=global
  wires:
  Sum/1 -> Heading_Compass/1, Scope8/1, To Workspace1/1, [Heading_Magnetometer_Noisy]
  Constant/1 -> Sum/1
  [Heading_Total_Wave_Control] -> Sum/2

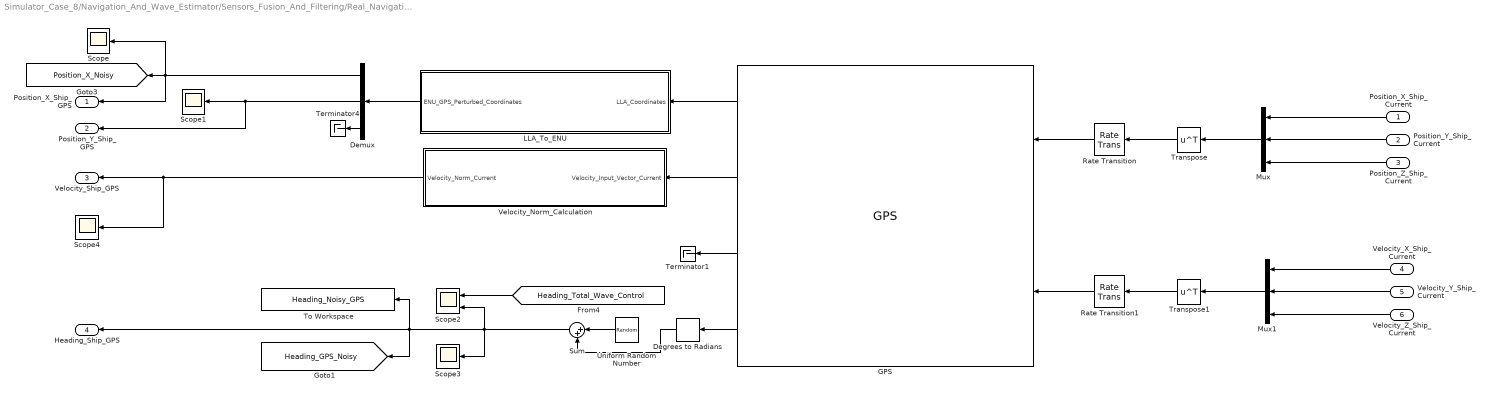
== system Simulator_Case_8/Navigation_And_Wave_Estimator/Sensors_Fusion_And_Filtering/Real_Navigation_Sensors_Extended_Kalman_Filter/GPS_Sensor ==
  Position_X_Ship_Current : Inport
  Position_Y_Ship_Current : Inport  Port=2
  Position_Z_Ship_Current : Inport  Port=3
  Velocity_X_Ship_Current : Inport  Port=4
  Velocity_Y_Ship_Current : Inport  Port=5
  Velocity_Z_Ship_Current : Inport  Port=6
  Degrees to Radians : simulink_extras/Transformations/Degrees to Radians
  Demux : Demux  Outputs=3
  GPS : sensorgpslib/GPS  DispRefFrame=ENU  PositionInputFormat=Local  ReferenceLocation=[43.059023, 3.002915 ,0]  HorizontalPositionAccuracy=2  VerticalPositionAccuracy=2  VelocityAccuracy=0.1  DecayFactor=0.999  SeedDouble=67  SimulateUsing=Interpreted execution
  LLA_To_ENU : MATLAB Function  TreatAsAtomicUnit=on  SystemSampleTime=Time_Period_Sampling
  Mux : Mux  Inputs=3
  Mux1 : Mux  Inputs=3
  Rate Transition : RateTransition  OutPortSampleTime=Time_Period_Sampling
  Rate Transition1 : RateTransition  OutPortSampleTime=Time_Period_Sampling
  Scope{,1,3..4} (4 alike) : Scope
  Scope2 : Scope  NumInputPorts=2
  Sum : Sum  Inputs=|++
  Terminator1 : Terminator
  Terminator4 : Terminator
  To Workspace : ToWorkspace  VariableName=Heading_Noisy_GPS  SaveFormat=Timeseries  SampleTime=Time_Period_Sampling
  Transpose : Math  Operator=transpose
  Transpose1 : Math  Operator=transpose
  Uniform Random Number : UniformRandomNumber  Minimum=-5*(pi/180)  Maximum=5*(pi/180)  SampleTime=Time_Period_Sampling
  Velocity_Norm_Calculation : MATLAB Function  TreatAsAtomicUnit=on
  Position_X_Ship_GPS : Outport
  Position_Y_Ship_GPS : Outport  Port=2
  Velocity_Ship_GPS : Outport  Port=3
  Heading_Ship_GPS : Outport  Port=4
  tag scope: Heading_GPS_Noisy=global, Position_X_Noisy=global
  wires:
  Demux/1 -> Scope/1, [Position_X_Noisy], Position_X_Ship_GPS/1
  Transpose1/1 -> Rate Transition1/1
  Velocity_Norm_Calculation/1(Velocity_Norm_Current) -> Scope4/1, Velocity_Ship_GPS/1
  Demux/2 -> Scope1/1, Position_Y_Ship_GPS/1
  Position_Z_Ship_Current/1 -> Mux/3
  Transpose/1 -> Rate Transition/1
  Position_X_Ship_Current/1 -> Mux/1
  GPS/1 -> LLA_To_ENU/1(LLA_Coordinates)
  Rate Transition1/1 -> GPS/2
  Velocity_X_Ship_Current/1 -> Mux1/1
  Demux/3 -> Terminator4/1
  LLA_To_ENU/1(ENU_GPS_Perturbed_Coordinates) -> Demux/1
  Mux/1 -> Transpose/1
  GPS/3 -> Terminator1/1
  GPS/4 -> Degrees to Radians/1
  Mux1/1 -> Transpose1/1
  [Heading_Total_Wave_Control] -> Scope2/1
  GPS/2 -> Velocity_Norm_Calculation/1(Velocity_Input_Vector_Current)
  Rate Transition/1 -> GPS/1
  Position_Y_Ship_Current/1 -> Mux/2
  Velocity_Y_Ship_Current/1 -> Mux1/2
  Velocity_Z_Ship_Current/1 -> Mux1/3
  Degrees to Radians/1 -> Sum/2
  Uniform Random Number/1 -> Sum/1
  Sum/1 -> Scope3/1, Scope2/2, Heading_Ship_GPS/1, [Heading_GPS_Noisy], To Workspace/1

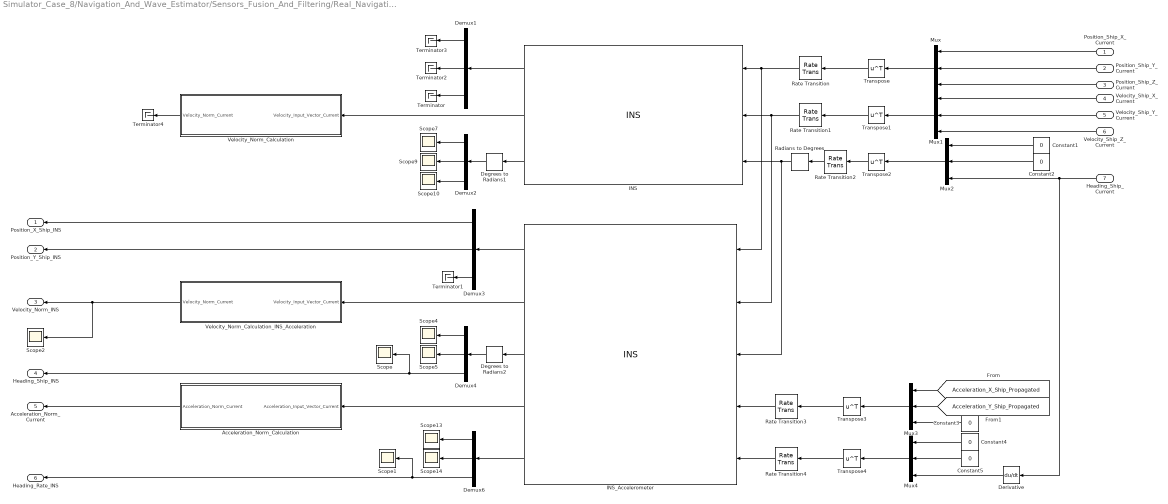
== system Simulator_Case_8/Navigation_And_Wave_Estimator/Sensors_Fusion_And_Filtering/Real_Navigation_Sensors_Extended_Kalman_Filter/INS_Sensor ==
  Position_Ship_X_Current : Inport
  Position_Ship_Y_Current : Inport  Port=2
  Position_Ship_Z_Current : Inport  Port=3
  Velocity_Ship_X_Current : Inport  Port=4
  Velocity_Ship_Y_Current : Inport  Port=5
  Velocity_Ship_Z_Current : Inport  Port=6
  Heading_Ship_Current : Inport  Port=7
  Acceleration_Norm_Calculation : MATLAB Function  TreatAsAtomicUnit=on
  Constant{1..5} (5 alike) : Constant  Value=0
  Degrees to Radians1 : simulink_extras/Transformations/Degrees to Radians
  Degrees to Radians2 : simulink_extras/Transformations/Degrees to Radians
  Demux{1..4,6} (5 alike) : Demux  Outputs=3
  Derivative : Derivative
  INS : sensorinslib/INS  MountingLocation=[0 0 0]  RollAccuracy=0.2  PitchAccuracy=0.2  YawAccuracy=0.5  PositionAccuracy=1  VelocityAccuracy=0.2  UseAccelAndAngVel=off  AccelerationAccuracy=0  AngularVelocityAccuracy=0  TimeInput=off  PositionErrorFactor=[0 0 0]  SeedDouble=67  SimulateUsing=Code generation
      settings: LibrarySourceBlock=mspsensorlib/INS
  INS_Accelerometer : sensorinslib/INS  MountingLocation=[0 0 0]  RollAccuracy=0.2  PitchAccuracy=0.2  YawAccuracy=0.5  PositionAccuracy=1  VelocityAccuracy=0.2  UseAccelAndAngVel=on  AccelerationAccuracy=0.02  AngularVelocityAccuracy=0.1  TimeInput=off  PositionErrorFactor=[0 0 0]  SeedDouble=67  SimulateUsing=Code generation
      settings: LibrarySourceBlock=mspsensorlib/INS
  Mux{,1..4} (5 alike) : Mux  Inputs=3
  Radians to Degrees : simulink_extras/Transformations/Radians to Degrees
  Rate Transition{,1..4} (5 alike) : RateTransition  OutPortSampleTime=Time_Period_Sampling
  Scope{,1..2,4..5,7,9..10,13..14} (10 alike) : Scope
  Terminator{,1..4} (5 alike) : Terminator
  Transpose{,1..4} (5 alike) : Math  Operator=transpose
  Velocity_Norm_Calculation : MATLAB Function  TreatAsAtomicUnit=on
  Velocity_Norm_Calculation_INS_Acceleration : MATLAB Function  TreatAsAtomicUnit=on
  Position_X_Ship_INS : Outport
  Position_Y_Ship_INS : Outport  Port=2
  Velocity_Norm_INS : Outport  Port=3
  Heading_Ship_INS : Outport  Port=4
  Acceleration_Norm_Current : Outport  Port=5
  Heading_Rate_INS : Outport  Port=6
  wires:
  Heading_Ship_Current/1 -> Derivative/1, Mux2/3
  Radians to Degrees/1 -> INS_Accelerometer/3, INS/3
  Position_Ship_X_Current/1 -> Mux/1
  Mux/1 -> Transpose/1
  Transpose/1 -> Rate Transition/1
  Velocity_Ship_Y_Current/1 -> Mux1/2
  Rate Transition2/1 -> Radians to Degrees/1
  Transpose2/1 -> Rate Transition2/1
  Constant1/1 -> Mux2/1
  INS/3 -> Degrees to Radians1/1
  Position_Ship_Y_Current/1 -> Mux/2
  Demux2/3 -> Scope10/1
  Demux2/1 -> Scope7/1
  INS/2 -> Velocity_Norm_Calculation/1(Velocity_Input_Vector_Current)
  Position_Ship_Z_Current/1 -> Mux/3
  Constant2/1 -> Mux2/2
  Velocity_Ship_X_Current/1 -> Mux1/1
  Demux2/2 -> Scope9/1
  Mux2/1 -> Transpose2/1
  Demux1/2 -> Terminator2/1
  Degrees to Radians1/1 -> Demux2/1
  Mux1/1 -> Transpose1/1
  INS/1 -> Demux1/1
  Rate Transition/1 -> INS_Accelerometer/1, INS/1
  Transpose1/1 -> Rate Transition1/1
  Rate Transition1/1 -> INS_Accelerometer/2, INS/2
  Velocity_Ship_Z_Current/1 -> Mux1/3
  Demux1/3 -> Terminator/1
  Transpose3/1 -> Rate Transition3/1
  Mux3/1 -> Transpose3/1
  Rate Transition3/1 -> INS_Accelerometer/4
  [Acceleration_X_Ship_Propagated] -> Mux3/1
  [Acceleration_Y_Ship_Propagated] -> Mux3/2
  Constant3/1 -> Mux3/3
  Constant4/1 -> Mux4/1
  Constant5/1 -> Mux4/2
  Derivative/1 -> Mux4/3
  Transpose4/1 -> Rate Transition4/1
  Rate Transition4/1 -> INS_Accelerometer/5
  Mux4/1 -> Transpose4/1
  INS_Accelerometer/1 -> Demux3/1
  Demux3/3 -> Terminator1/1
  INS_Accelerometer/2 -> Velocity_Norm_Calculation_INS_Acceleration/1(Velocity_Input_Vector_Current)
  INS_Accelerometer/3 -> Degrees to Radians2/1
  Demux4/1 -> Scope4/1
  Degrees to Radians2/1 -> Demux4/1
  Demux4/3 -> Scope/1, Heading_Ship_INS/1
  Demux4/2 -> Scope5/1
  INS_Accelerometer/5 -> Demux6/1
  Demux6/1 -> Scope13/1
  Demux6/2 -> Scope14/1
  Demux6/3 -> Scope1/1, Heading_Rate_INS/1
  Acceleration_Norm_Calculation/1(Acceleration_Norm_Current) -> Acceleration_Norm_Current/1
  Demux3/1 -> Position_X_Ship_INS/1
  Demux3/2 -> Position_Y_Ship_INS/1
  Velocity_Norm_Calculation_INS_Acceleration/1(Velocity_Norm_Current) -> Scope2/1, Velocity_Norm_INS/1
  INS_Accelerometer/4 -> Acceleration_Norm_Calculation/1(Acceleration_Input_Vector_Current)
  Demux1/1 -> Terminator3/1
  Velocity_Norm_Calculation/1(Velocity_Norm_Current) -> Terminator4/1

== matlab function Simulator_Case_8/Navigation_And_Wave_Estimator/Wave_Estimation_Kalman_Filter/Wave_Heading_Estimation ==
  data: Heading_Total_Observed_Current input; Rudder_Angle_Commanded_Current input; Wave_Pulsation_Estimated input; Damping_Wave_Estimated input; Time_Current input; Time_Constant_Ship input; Gain_Ship input; Time_Sampling input; Noise_For_Heading_wave input; Heading_Rate_Wave_Estimated_Current output; Heading_Wave_Estimated_Current output; Heading_Low_Frequency_Estimated_Current output; Heading_Rate_Estimated_Current output; Bias_Estimated_Current output; Covariance_Aposteriori_Estimate output; Torque_Wind_Estimated_Input input; Inertia_Ship_Vertical input; Wave_Pulsation_Identified input; Heading_Rate_Estimated_Current_Navigation input; Length_Ship_Current input; Density_Water_Current input; Drag_Coefficient_Current input; Draft_Depth_Current input; Longeron_Area_Current input; Mass_Of_The_Ship_Current input; Velocity_Current_Estimated input
function [Heading_Rate_Wave_Estimated_Current,...
          Heading_Wave_Estimated_Current,...
          Heading_Low_Frequency_Estimated_Current,...
          Heading_Rate_Estimated_Current,...
          Bias_Estimated_Current,...
          Covariance_Aposteriori_Estimate]= Kalman_Filter_Wave_Estimation(Heading_Total_Observed_Current,...
                                                                          Rudder_Angle_Commanded_Current,...
                                                                          Wave_Pulsation_Estimated,...
                                                                          Damping_Wave_Estimated,...
                                                                          Time_Current,...
                                                                          Time_Constant_Ship,...
                                                                          Gain_Ship,...
                                                                          Time_Sampling,...
                                                                          Noise_For_Heading_wave,...
                                                                          Torque_Wind_Estimated_Input,...
                                                                          Inertia_Ship_Vertical,...
                                                                          Wave_Pulsation_Identified,...
                                                                          Heading_Rate_Estimated_Current_Navigation,...
                                                                          Length_Ship_Current,...
                                                                          Density_Water_Current,...
                                                                          Drag_Coefficient_Current,...
                                                                          Draft_Depth_Current,...
                                                                          Longeron_Area_Current,...
                                                                          Mass_Of_The_Ship_Current,...
                                                                          Velocity_Current_Estimated)

% Time constant and ship static gain evolution in function of the velocity
% to be computed:
Is_Estimation_Ship_Parameters = 1;
if Is_Estimation_Ship_Parameters
    [Static_Gain,Time_Constant] = Static_Gain_Time_Constant_Varying_Velocity(Velocity_Current_Estimated,... % Considered to be the cleanest.
                                                                             Length_Ship_Current,...
                                                                             Density_Water_Current,...
                                                                             Drag_Coefficient_Current,...
                                                                             Draft_Depth_Current,...
                                                                             Longeron_Area_Current,...
                                                                             Mass_Of_The_Ship_Current);
else
    Static_Gain = Gain_Ship;
    Time_Constant = Time_Constant_Ship;
end

% Online Wave Observer Kalman algorithm for better wave high frequency
% filtering:
Is_Discretization_Euler = 1;
if Is_Discretization_Euler
    [Heading_Rate_Wave_Estimated_Current,...
     Heading_Wave_Estimated_Current,...
     Heading_Low_Frequency_Estimated_Current,...
     Heading_Rate_Estimated_Current,...
     Bias_Estimated_Current,...
     Covariance_Aposteriori_Estimate] = Kalman_Observer_Wave_Estimation_Dynamics(Heading_Total_Observed_Current,...
                                                                                 Rudder_Angle_Commanded_Current,...
                                                                                 Wave_Pulsation_Estimated,...
                                                                                 Damping_Wave_Estimated,...
                                                                                 Time_Current,...
                                                                                 Time_Constant,...
                                                                                 Static_Gain,...
                                                                                 Time_Sampling,...
                                                                                 Noise_For_Heading_wave,...
                                                                                 Torque_Wind_Estimated_Input,...
                                                                                 Inertia_Ship_Vertical,...
                                                                                 Wave_Pulsation_Identified,...
                                                                                 Heading_Rate_Estimated_Current_Navigation);
else % Exponential matrix discretization:
    [Heading_Rate_Wave_Estimated_Current,...
     Heading_Wave_Estimated_Current,...
     Heading_Low_Frequency_Estimated_Current,...
     Heading_Rate_Estimated_Current,...
     Bias_Estimated_Current,...
     Covariance_Aposteriori_Estimate] = Kalman_Observer_Wave_Estimation_Discretization(Heading_Total_Observed_Current,...
                                                                                       Rudder_Angle_Commanded_Current,...
                                                                                       Wave_Pulsation_Estimated,...
                                                                                       Damping_Wave_Estimated,...
                                                                                       Time_Current,...
                                                                                       Time_Constant,...
                                                                                       Static_Gain,...
                                                                                       Time_Sampling,...
                                                                                       Noise_For_Heading_wave,...
                                                                                       Torque_Wind_Estimated_Input,...
                                                                                       Inertia_Ship_Vertical,...
                                                                                       Wave_Pulsation_Identified,...
                                                                                       Heading_Rate_Estimated_Current_Navigation);


end

== matlab function Simulator_Case_8/Navigation_And_Wave_Estimator/Sensors_Fusion_And_Filtering/Real_Navigation_Sensors_Extended_Kalman_Filter/GPS_Sensor/LLA_To_ENU ==
  data: LLA_Coordinates input; ENU_GPS_Perturbed_Coordinates output
function ENU_GPS_Perturbed_Coordinates = Conversion_LLA_To_ENU(LLA_Coordinates)

% Reference point:
Reference_Point_Port_Mahon = [43.059023,3.002915,0];
Semi_Major_Axis = 6378137.0;
Flattening = 1/298.25;

% This function serves as a mean to convert LLA coordinates to ENU
% coordinates:
ENU_GPS_Perturbed_Coordinates = LLA_To_ENU(LLA_Coordinates(1),LLA_Coordinates(2),LLA_Coordinates(3),...
                                           Reference_Point_Port_Mahon(1),Reference_Point_Port_Mahon(2),...
                                           Reference_Point_Port_Mahon(3),Semi_Major_Axis,Flattening);


end

== matlab function Simulator_Case_8/Navigation_And_Wave_Estimator/Sensors_Fusion_And_Filtering/Real_Navigation_Sensors_Extended_Kalman_Filter/GPS_Sensor/Velocity_Norm_Calculation ==
  data: Velocity_Input_Vector_Current input; Velocity_Norm_Current output
function Velocity_Norm_Current = Velocity_Norm(Velocity_Input_Vector_Current)

% Norm calculation:
Velocity_Norm_Current = sqrt(Velocity_Input_Vector_Current(1)^2 + Velocity_Input_Vector_Current(2)^2 + Velocity_Input_Vector_Current(3)^2);

end
